simulink model "pendulum_mode"  (R2017a)
settings: Solver=FixedStepAuto  StartTime=0.0  StopTime=10.0  FixedStep=0.01  RelTol=1e-3
values from neighbouring files (symbols this model uses):
  c = -X(1)*(m*l^2)    [derivative_example.m]
  g = 9.81    [derivative_example.m]
  l = -g/X(2)    [derivative_example.m]
  m = 0.2    [derivative_example.m]
settings Model: Creator=Patrick  LastModifiedBy=Patrick

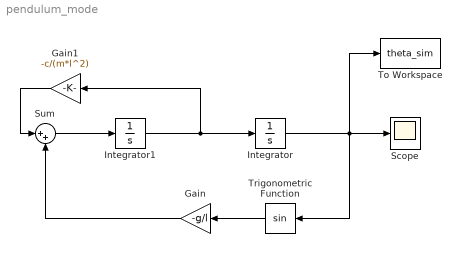
== system pendulum_mode ==
  Gain : Gain  Gain=-g/l
  Gain1 : Gain  Gain=-c/(m*l^2)
  Integrator : Integrator  InitialCondition=1.104300000000000
  Integrator1 : Integrator
  Scope : Scope
  Sum : Sum  Inputs=|++
  To Workspace : ToWorkspace  VariableName=theta_sim  SampleTime=-1
  Trigonometric Function : Trigonometry
  wires:
  Integrator/1 -> To Workspace/1, Scope/1, Trigonometric Function/1
  Integrator1/1 -> Integrator/1, Gain1/1
  Trigonometric Function/1 -> Gain/1
  Sum/1 -> Integrator1/1
  Gain1/1 -> Sum/1
  Gain/1 -> Sum/2
